simulink model "bicyclemodel"  (R2015a)
settings: Solver=ode45  StartTime=0.0  StopTime=10.0  RelTol=1e-3
undefined symbols (not defined in the file): Df, L1, v
settings Model: Creator=Sara  LastModifiedBy=Sara

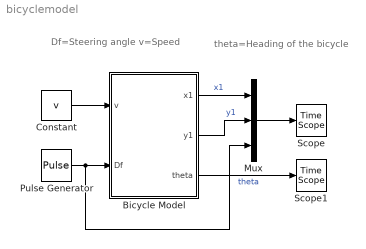
== system bicyclemodel ==
  note: theta=Heading of the bicycle
  note: Df=Steering angle
      | v=Speed
  Bicycle Model : Subsystem
  Constant : Constant  Value=v
  Mux : Mux  Inputs=3
  Pulse Generator : DiscretePulseGenerator  PulseType=Time based  Amplitude=Df  Period=10  PulseWidth=5
  Scope : TimeScope
  Scope1 : TimeScope
  wires:
  Constant/1 -> Bicycle Model/1(v)
  Bicycle Model/1(x1) -> Mux/1  "x1"
  Bicycle Model/2(y1) -> Mux/2  "y1"
  Mux/1 -> Scope/1
  Bicycle Model/3(theta) -> Scope1/1  "theta"
  Pulse Generator/1 -> Mux/3, Bicycle Model/2(Df)

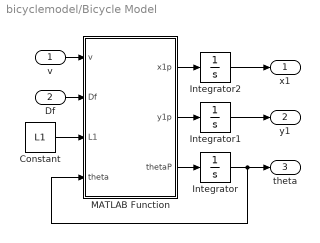
== system bicyclemodel/Bicycle Model ==
  v : Inport
  Df : Inport  Port=2
  Constant : Constant  Value=L1
  Integrator : Integrator
  Integrator1 : Integrator
  Integrator2 : Integrator
  MATLAB Function : MATLAB Function  TreatAsAtomicUnit=on
  x1 : Outport
  y1 : Outport  Port=2
  theta : Outport  Port=3
  wires:
  MATLAB Function/1(x1p) -> Integrator2/1
  MATLAB Function/3(thetaP) -> Integrator/1
  Integrator1/1 -> y1/1
  v/1 -> MATLAB Function/1(v)
  Integrator2/1 -> x1/1
  Df/1 -> MATLAB Function/2(Df)
  Integrator/1 -> MATLAB Function/4(theta), theta/1
  MATLAB Function/2(y1p) -> Integrator1/1
  Constant/1 -> MATLAB Function/3(L1)

== matlab function bicyclemodel/Bicycle Model/MATLAB Function ==
  data: x1p output; y1p output; v input; thetaP output; Df input; L1 input; theta input
function [x1p,y1p,thetaP] = fcn(v,Df,L1,theta)
%Rotation rate equation
thetaP=(v*sin(Df))/L1;

x1p=v*cos(theta+Df);
y1p=v*sin(theta+Df);
